simulink model "SimscapeCrane_ClosedLoop"  (R2016a)
settings: Solver=ode15s  StartTime=0.0  StopTime=60  RelTol=1e-3
model workspace: external: MAT-File workspace.mat (data not in the file)
values from neighbouring files (symbols this model uses):
  m = 0.47    [CraneParameters.mat]
  MR = 1.71    [CraneParameters.mat]
  N = ceil(Tf/Ts)    [Best_Shape_1_NO_ALGO_CHANGES.m]    (also in Best_Shape_2_NO_ALGO_CHANGES.m; FunctionTemplate_S1.m; FunctionTemplate_S1_OLD.m; FunctionTemplate_S2.m)
  Ts = 1/20    (= 0.05)    [Best_Shape_1_NO_ALGO_CHANGES.m]    (also in Best_Shape_2_NO_ALGO_CHANGES.m; FunctionTemplate_S1.m; FunctionTemplate_S1_OLD.m; FunctionTemplate_S2.m)
  xRange = [0 0.52]    [cw3_part4.m]    (also in cw3_soft_constraints.m)
  xZero = xRange(1)    [cw3_soft_constraints.m]    (also in testMyDesign.m = startingPoint(1,1); testMyDesign_Linear.m = startingPoint(1,1))
  yRange = [0 0.52]    [cw3_part4.m]    (also in cw3_soft_constraints.m = [0 0.62])
  yZero = yRange(1)    [cw3_soft_constraints.m]    (also in testMyDesign.m = startingPoint(1,2); testMyDesign_Linear.m = startingPoint(1,2))
undefined symbols (not defined in the file or in its folder): TxBreak, TxCoulomb, TxVisc, TyBreak, TyCoulomb, TzBreak, TzCoulomb, X, Y, Z, zRange, zZero
undefined symbols (not defined in the file): M, param, TorqueMultX, TorqueMultY, TorqueMultZ, TxTrans, TyTrans, TyVisc, TzTrans, TzVisc
libraries: sm_lib x146, fl_lib x62, nesl_utility x24, elec_lib x9, simulink x6, sm_double_wishbone_suspension_lib x4, aerolibtransform2 x1
(part 1 of 14)
settings Model: Creator=jsustare  LastModifiedBy=vinay
settings SolverCC: MaxConsecutiveMinStep=10
settings DataIOCC: SaveFormat=StructureWithTime
settings DebuggingCC: AllowSymbolicDim=off
settings ModelReferenceCC: PropagateSignalLabelsOutOfModel=off
settings GRTTargetCC: GeneratePreprocessorConditionals=Use local settings
settings ConfigurationSet: Description=SimMechanics 2G

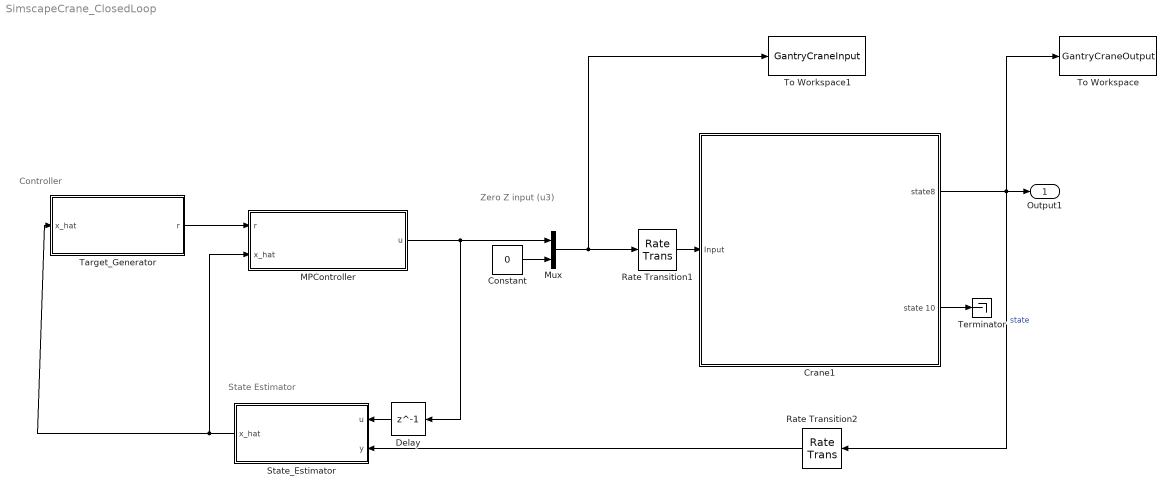
== system SimscapeCrane_ClosedLoop ==
  note: Controller
  note: Zero Z input (u3)
  note: State Estimator
  Constant : Constant  Value=0
  Crane1 : Subsystem  mask{penduMass=m, cartMass=M, MR=MR, xRange=xRange, yRange=yRange, zRange=zRange, xZero=xZero, yZero=yZero, zZero=zZero, TxBreak=TxBreak, TxCoulomb=TxCoulomb, TxVisc=TxVisc, TxTrans=TxTrans, TyBreak=TyBreak, TyCoulomb=TyCoulomb, TyVisc=TyVisc, TyTrans=TyTrans, TzBreak=TzBreak, TzCoulomb=TzCoulomb, TzVisc=TzVisc, TzTrans=TzTrans, Ux=TorqueMultX, Uy=TorqueMultY, Uz=TorqueMultZ}
      mask prompts: penduMass "Pendulum Mass (Kg)"; cartMass "Mass of the cart (Kg)"; MR "Mass of the rail (Kg)"; TxBreak "BreakAwayFriction"; TxCoulomb "Coulomb Friction"; TxVisc "Viscous friction"; TxTrans "Transition coeff"; TyBreak "BreakAwayFriction"; TyCoulomb "Coulomb Friction"; TyVisc "Viscous friction"; TyTrans "Transition coeff"; TzBreak "BreakAwayFriction"; TzCoulomb "Coulomb Friction"; TzVisc "Viscous friction"; TzTrans "Transition coeff"; Ux "Rail motor multiplier (X)"; Uy "Cart motor multiplier (Y)"; Uz "String motor multiplier (Z)"
      mask init:
      | %mass lowSat
      | penduMass=max(penduMass,1e-3);
      | cartMass=max(cartMass,1e-3);
      | MR=max(MR,1e-3);
      | 
      | %zeros saturated
      | xZero=max(xZero,xRange(1));
      | xZero=min(xZero,xRange(2));
      | 
      | yZero=max(yZero,yRange(1));
      | yZero=min(yZero,yRange(2));
      | 
      | zZero=max(zZero,zRange(1));
      | zZero=min(zZero,zRange(2));
      mask DialogControl DescGroupVar Prompt: 3D Crane Simscape model
      mask Display:
